simulink model "IEEE123_4subsystem"  (R2022b)
settings: Solver=ode4  StartTime=0.0  StopTime=inf  FixedStep=Ts  MaxStep=1e-4  RelTol=1e-3
PreLoadFcn:
  | Ts = 50e-6;
PostLoadFcn:
  | Ts = 50e-6;
InitFcn:
  | %%%%%%%%%%%%%%%%%%%%%%%%
  | % Simulation data for the IEEE 123 Node Test Feeder model
  | %%%%%%%%%%%%%%%%%%%%%%%
  | 
  | % miles/km
  | mi2km = 1.60934;
  | 
  | % feet to km
  | ft2km = 0.0003048;
  | 
  | % microsiemens to Farads
  | ms2F = 1/2/pi/60*1e-6;
  | 
  | %% Configuration 1 - series reactance - ohm/mile
  | 
  | R_1 = [0.4576 0.1560 0.1535;0.1560 0.4666 0.1580;0.1535 0.1580 0.4615];
  | X_1 = [1.0780 0.5017 0.3849;0.5017 1.0482 0.4236;0.3849 0.4236 1.0651];
  | 
  | % charging susceptance - microsiemens/mile
  | 
  | B_1 = [5.6765 -1.8319 -0.6982;-1.8319 5.9809 -1.1645;-0.6982 -1.1645 5.3971];
  | 
  | % convert for SPS
  | 
  | R_1 = R_1/mi2km;
  | 
  | Rs_1=(R_1(1,1)+R_1(2,2)+R_1(3,3))/3;
  | Rm_1=(R_1(1,2)+R_1(1,3)+R_1(2,3))/3;
  | R1_1=Rs_1-Rm_1;
  | R0_1=Rs_1+2*Rm_1;
  | 
  | L_1 = X_1/mi2km/2/pi/60;
  | 
  | Ls_1=(L_1(1,1)+L_1(2,2)+L_1(3,3))/3;
  | Lm_1=(L_1(1,2)+L_1(1,3)+L_1(2,3))/3;
  | L1_1=Ls_1-Lm_1;
  | L0_1=Ls_1+2*Lm_1;
  | 
  | C_1 = B_1/mi2km*ms2F;
  | 
  | Cs_1=(C_1(1,1)+C_1(2,2)+C_1(3,3))/3;
  | Cm_1=(C_1(1,2)+C_1(1,3)+C_1(2,3))/3;
  | C1_1=Cs_1-Cm_1;
  | C0_1=Cs_1+2*Cm_1;
  | 
  | 
  | %% Configuration 2 - series reactance - ohm/mile
  | 
  | R_2 = [0.4666 0.1580 0.1560;0.1580 0.4615 0.1535;0.1560 0.1535 0.4576];
  | X_2 = [1.0482 0.4236 0.5017;0.4236 1.0651 0.3849;0.5017 0.3849 1.0780];
  | 
  | % charging susceptance - microsiemens/mile
  | 
  | B_2 = [5.9809 -1.1645 -1.8319;-1.1645 5.3971 -0.6982;-1.8319 -0.6982 5.6765];
  | 
  | % convert for SPS
  | 
  | R_2 = R_2/mi2km;
  | 
  | Rs_2=(R_2(1,1)+R_2(2,2)+R_2(3,3))/3;
  | ... (+341 lines)
undefined symbols (not defined in the file): D1, Delta, find_system, I, Left, MOV_segment9, powergui, Right, type, V, X
libraries: spsGroundLib x242, spsThreePhaseVIMeasurementLib x134, spsSeriesRLCBranchLib x107, spsSeriesRLCLoadLib x83, spsPiSectionLineLib x61, spsThreePhasePISectionLineLib x60, spsVoltageMeasurementLib x52, spsDCVoltageSourceLib x36, ssn_lib x28, artemis x24, spsACCurrentSourceLib x18, spsOnDelayLib x18
(part 14 of 15)

== system IEEE123_4subsystem/SS_123p1/Regulator 4/Single Phase SVR_B/Transformer with Taps/SSN OLTC xfo v2/conn_down_d ==
  b2 : PMIOPort  Side=Right
  b1 : PMIOPort  Port=2  Side=Left
  connections:
  b1/RConn1 -- b2/RConn1

== system IEEE123_4subsystem/SS_123p1/Regulator 4/Single Phase SVR_B/Transformer with Taps/SSN OLTC xfo v2/conn_up_c ==
  b2 : PMIOPort  Side=Right
  b1 : PMIOPort  Port=2  Side=Left
  connections:
  b1/RConn1 -- b2/RConn1

== system IEEE123_4subsystem/SS_123p1/Regulator 4/Single Phase SVR_B/Transformer with Taps/SSN OLTC xfo v2/conn_up_d ==
  b2 : PMIOPort  Side=Right
  b1 : PMIOPort  Port=2  Side=Left
  connections:
  b1/RConn1 -- b2/RConn1

== system IEEE123_4subsystem/SS_123p1/Regulator 4/Single Phase SVR_B/Voltage Regulator Control/Tap Changer Control/Determine tap position ==
  NewTap : Inport
  Trigger : TriggerPort  VariantControl=Variant
  Memory : Memory  InitialCondition=InitialPosition  InheritSampleTime=on
  Saturation : Saturate  UpperLimit=MinMaxTap(2)  LowerLimit=MinMaxTap(1)
  Sum : Sum  Inputs=|++  SaturateOnIntegerOverflow=on
  TapNo : Outport  InitialOutput=InitialPosition  VectorParamsAs1DForOutWhenUnconnected=off
  wires:
  Saturation/1 -> Memory/1, TapNo/1
  Memory/1 -> Sum/2
  Sum/1 -> Saturation/1
  NewTap/1 -> Sum/1

== system IEEE123_4subsystem/SS_123p1/Regulator 4/Single Phase SVR_B/Voltage Regulator Control/Tap Changer Control/Edge Detector ==
  note: Edge or Slope Detector
  In : Inport
  Constant1 : Constant  Value=model
  Demux : Demux  Outputs=2
      settings: DisplayOption=none
  Logical Operator1 : Logic  Operator=OR
  Memory : Memory  InitialCondition=ic  LinearizeAsDelay=on
  Multiport Switch : MultiPortSwitch  InputSameDT=off
  NEGATIVE Edge : Subsystem  TreatAsAtomicUnit=on
  POSITIVE Edge : Subsystem  TreatAsAtomicUnit=on
  either edge : Constant  Value=[1 1]
  neg. edge : Constant  Value=[0 1]
  pos. edge : Constant  Value=[1 0]
  Out : Outport  VectorParamsAs1DForOutWhenUnconnected=off
  wires:
  Logical Operator1/1 -> Out/1
  NEGATIVE Edge/1(OUT) -> Logical Operator1/2
  POSITIVE Edge/1(OUT) -> Logical Operator1/1
  Memory/1 -> POSITIVE Edge/2(IN previous), NEGATIVE Edge/2(IN previous)
  In/1 -> POSITIVE Edge/1(IN), NEGATIVE Edge/1(IN), Memory/1
  pos. edge/1 -> Multiport Switch/2
  neg. edge/1 -> Multiport Switch/3
  Constant1/1 -> Multiport Switch/1
  Multiport Switch/1 -> Demux/1
  Demux/1 -> POSITIVE Edge/Enable
  Demux/2 -> NEGATIVE Edge/Enable
  either edge/1 -> Multiport Switch/4

== system IEEE123_4subsystem/SS_123p1/Regulator 4/Single Phase SVR_C/Transformer with Taps/SSN OLTC xfo v2/DC source_a ==
  I1A_V : spsDCVoltageSourceLib/DC Voltage Source  Amplitude=0  Measurements=None
  Conn1 : PMIOPort  Side=Left
  Conn2 : PMIOPort  Port=2  Side=Right
  connections:
  Conn1/RConn1 -- I1A_V/LConn1
  Conn2/RConn1 -- I1A_V/RConn1

== system IEEE123_4subsystem/SS_123p1/Regulator 4/Single Phase SVR_C/Transformer with Taps/SSN OLTC xfo v2/DC source_b ==
  I1B_V : spsDCVoltageSourceLib/DC Voltage Source  Amplitude=0  Measurements=None
  Conn3 : PMIOPort  Side=Left
  Conn4 : PMIOPort  Port=2  Side=Right
  connections:
  Conn4/RConn1 -- I1B_V/RConn1
  Conn3/RConn1 -- I1B_V/LConn1

== system IEEE123_4subsystem/SS_123p1/Regulator 4/Single Phase SVR_C/Transformer with Taps/SSN OLTC xfo v2/DC source_c ==
  I1C_V : spsDCVoltageSourceLib/DC Voltage Source  Amplitude=0  Measurements=None
  Conn1 : PMIOPort  Side=Left
  Conn2 : PMIOPort  Port=2  Side=Right
  connections:
  Conn2/RConn1 -- I1C_V/RConn1
  Conn1/RConn1 -- I1C_V/LConn1

== system IEEE123_4subsystem/SS_123p1/Regulator 4/Single Phase SVR_C/Transformer with Taps/SSN OLTC xfo v2/DC source_d ==
  I1D_V : spsDCVoltageSourceLib/DC Voltage Source  Amplitude=0  Measurements=None
  Conn3 : PMIOPort  Side=Left
  Conn4 : PMIOPort  Port=2  Side=Right
  connections:
  Conn3/RConn1 -- I1D_V/LConn1
  Conn4/RConn1 -- I1D_V/RConn1

== system IEEE123_4subsystem/SS_123p1/Regulator 4/Single Phase SVR_C/Transformer with Taps/SSN OLTC xfo v2/SSS-SM equations ==
  A : Inport
  B : Inport  Port=2
  C : Inport  Port=3
  u : Inport  Port=4
  Flux0 : Inport  Port=5
  Bphic : Inport  Port=6
  be : Inport  Port=7
  Constant : Constant
  Discretize : Subsystem
  Product{1..3,5..6} (5 alike) : Product  Multiplication=Matrix(*)  SaturateOnIntegerOverflow=on  OutDataTypeStr=Inherit: Same as first input
  Sum1 : Sum  Inputs=-+  SaturateOnIntegerOverflow=on
  Sum2 : Sum  Inputs=+++  SaturateOnIntegerOverflow=on
  Sum3 : Sum  SaturateOnIntegerOverflow=on
  mult1 : Product
  u5 : Constant  Value=eye(3,3)
  z-1 : UnitDelay  SampleTime=Ts  HasFrameUpgradeWarning=on
  Y : Outport  VectorParamsAs1DForOutWhenUnconnected=off
  Ihist : Outport  Port=2  VectorParamsAs1DForOutWhenUnconnected=off
  x : Outport  Port=3  VectorParamsAs1DForOutWhenUnconnected=off
  wires:
  u5/1 -> Discretize/3(Unity)
  Product2/1 -> Y/1
  A/1 -> Discretize/1(Ac)
  B/1 -> Discretize/2(Bc)
  C/1 -> Product2/1, Product6/1
  Product6/1 -> Ihist/1
  Product5/1 -> Sum3/2, mult1/1
  Product3/1 -> Sum2/1
  Sum3/1 -> Product3/2, x/1  "new_x"
  Sum2/1 -> z-1/1, Product6/2
  Discretize/1(Ad) -> Product3/1
  u/1 -> Product5/2
  z-1/1 -> Sum3/1
  Discretize/2(Bd) -> Product5/1, Product2/2
  Discretize/3(Bdin) -> Product1/1
  Product1/1 -> Sum2/3
  Flux0/1 -> Product1/2
  Bphic/1 -> Discretize/4(Bphic)
  Constant/1 -> Sum1/2
  mult1/1 -> Sum2/2
  Sum1/1 -> mult1/2  "=1 if trapeze           =0 if BE"
  be/1 -> Discretize/5(be), Sum1/1

== system IEEE123_4subsystem/SS_123p1/Regulator 4/Single Phase SVR_C/Transformer with Taps/SSN OLTC xfo v2/Update Matrix L ==
  k : Inport
  L2 : Inport  Port=2
  Lin : Inport  Port=3
  "L2->(2,2) " : Assignment  NumberOfDimensions=2  IndexOptions=Index vector (dialog),Index vector (dialog)  Indices=[2],[2]  OutputSizes=1,1
  k->(2,3) : Assignment  NumberOfDimensions=2  IndexOptions=Index vector (dialog),Index vector (dialog)  Indices=[2],[3]  OutputSizes=1,1
  L : Outport  VectorParamsAs1DForOutWhenUnconnected=off
  wires:
  "L2->(2,2) "/1 -> L/1
  L2/1 -> "L2->(2,2) "/2
  Lin/1 -> k->(2,3)/1
  k/1 -> k->(2,3)/2
  k->(2,3)/1 -> "L2->(2,2) "/1

== system IEEE123_4subsystem/SS_123p1/Regulator 4/Single Phase SVR_C/Transformer with Taps/SSN OLTC xfo v2/Update Matrix R ==
  R2 : Inport
  Rin : Inport  Port=2
  k : Inport  Port=3
  Rcore : Inport  Port=4
  Rcore/Lcore : Inport  Port=5
  "-R2->(2,2) " : Assignment  NumberOfDimensions=2  IndexOptions=Index vector (dialog),Index vector (dialog)  Indices=[2],[2]  OutputSizes=1,1
  -Rm/Lm->(3,3) : Assignment  NumberOfDimensions=2  IndexOptions=Index vector (dialog),Index vector (dialog)  Indices=3,3  OutputSizes=1,1
  Gain : Gain  Gain=-1
  Gain1 : Gain  Gain=-1
  Product1 : Product  RndMeth=Zero
  kRm->(3,2) : Assignment  NumberOfDimensions=2  IndexOptions=Index vector (dialog),Index vector (dialog)  Indices=3,2  OutputSizes=1,1
  R : Outport  VectorParamsAs1DForOutWhenUnconnected=off
  wires:
  "-R2->(2,2) "/1 -> kRm->(3,2)/1
  R2/1 -> Gain/1
  Rin/1 -> "-R2->(2,2) "/1
  Gain/1 -> "-R2->(2,2) "/2
  k/1 -> Product1/2
  Product1/1 -> kRm->(3,2)/2
  kRm->(3,2)/1 -> -Rm/Lm->(3,3)/1
  -Rm/Lm->(3,3)/1 -> R/1
  Rcore/1 -> Product1/1
  Gain1/1 -> -Rm/Lm->(3,3)/2
  Rcore/Lcore/1 -> Gain1/1

== system IEEE123_4subsystem/SS_123p1/Regulator 4/Single Phase SVR_C/Transformer with Taps/SSN OLTC xfo v2/conn_down_c ==
  b2 : PMIOPort  Side=Right
  b1 : PMIOPort  Port=2  Side=Left
  connections:
  b1/RConn1 -- b2/RConn1

== system IEEE123_4subsystem/SS_123p1/Regulator 4/Single Phase SVR_C/Transformer with Taps/SSN OLTC xfo v2/conn_down_d ==
  b2 : PMIOPort  Side=Right
  b1 : PMIOPort  Port=2  Side=Left
  connections:
  b1/RConn1 -- b2/RConn1

== system IEEE123_4subsystem/SS_123p1/Regulator 4/Single Phase SVR_C/Transformer with Taps/SSN OLTC xfo v2/conn_up_c ==
  b2 : PMIOPort  Side=Right
  b1 : PMIOPort  Port=2  Side=Left
  connections:
  b1/RConn1 -- b2/RConn1

== system IEEE123_4subsystem/SS_123p1/Regulator 4/Single Phase SVR_C/Transformer with Taps/SSN OLTC xfo v2/conn_up_d ==
  b2 : PMIOPort  Side=Right
  b1 : PMIOPort  Port=2  Side=Left
  connections:
  b1/RConn1 -- b2/RConn1

== system IEEE123_4subsystem/SS_123p1/Regulator 4/Single Phase SVR_C/Voltage Regulator Control/Tap Changer Control/Determine tap position ==
  NewTap : Inport
  Trigger : TriggerPort  VariantControl=Variant
  Memory : Memory  InitialCondition=InitialPosition  InheritSampleTime=on
  Saturation : Saturate  UpperLimit=MinMaxTap(2)  LowerLimit=MinMaxTap(1)
  Sum : Sum  Inputs=|++  SaturateOnIntegerOverflow=on
  TapNo : Outport  InitialOutput=InitialPosition  VectorParamsAs1DForOutWhenUnconnected=off
  wires:
  Saturation/1 -> Memory/1, TapNo/1
  Memory/1 -> Sum/2
  Sum/1 -> Saturation/1
  NewTap/1 -> Sum/1

== system IEEE123_4subsystem/SS_123p1/Regulator 4/Single Phase SVR_C/Voltage Regulator Control/Tap Changer Control/Edge Detector ==
  note: Edge or Slope Detector
  In : Inport
  Constant1 : Constant  Value=model
  Demux : Demux  Outputs=2
      settings: DisplayOption=none
  Logical Operator1 : Logic  Operator=OR
  Memory : Memory  InitialCondition=ic  LinearizeAsDelay=on
  Multiport Switch : MultiPortSwitch  InputSameDT=off
  NEGATIVE Edge : Subsystem  TreatAsAtomicUnit=on
  POSITIVE Edge : Subsystem  TreatAsAtomicUnit=on
  either edge : Constant  Value=[1 1]
  neg. edge : Constant  Value=[0 1]
  pos. edge : Constant  Value=[1 0]
  Out : Outport  VectorParamsAs1DForOutWhenUnconnected=off
  wires:
  Logical Operator1/1 -> Out/1
  NEGATIVE Edge/1(OUT) -> Logical Operator1/2
  POSITIVE Edge/1(OUT) -> Logical Operator1/1
  Memory/1 -> POSITIVE Edge/2(IN previous), NEGATIVE Edge/2(IN previous)
  In/1 -> POSITIVE Edge/1(IN), NEGATIVE Edge/1(IN), Memory/1
  pos. edge/1 -> Multiport Switch/2
  neg. edge/1 -> Multiport Switch/3
  Constant1/1 -> Multiport Switch/1
  Multiport Switch/1 -> Demux/1
  Demux/1 -> POSITIVE Edge/Enable
  Demux/2 -> NEGATIVE Edge/Enable
  either edge/1 -> Multiport Switch/4

== system IEEE123_4subsystem/SS_123p2/Regulator3/Single Phase SVR_A/Transformer with Taps/SSN OLTC xfo v2/DC source_a ==
  I1A_V : spsDCVoltageSourceLib/DC Voltage Source  Amplitude=0  Measurements=None
  Conn1 : PMIOPort  Side=Left
  Conn2 : PMIOPort  Port=2  Side=Right
  connections:
  Conn1/RConn1 -- I1A_V/LConn1
  Conn2/RConn1 -- I1A_V/RConn1

== system IEEE123_4subsystem/SS_123p2/Regulator3/Single Phase SVR_A/Transformer with Taps/SSN OLTC xfo v2/DC source_b ==
  I1B_V : spsDCVoltageSourceLib/DC Voltage Source  Amplitude=0  Measurements=None
  Conn3 : PMIOPort  Side=Left
  Conn4 : PMIOPort  Port=2  Side=Right
  connections:
  Conn4/RConn1 -- I1B_V/RConn1
  Conn3/RConn1 -- I1B_V/LConn1

== system IEEE123_4subsystem/SS_123p2/Regulator3/Single Phase SVR_A/Transformer with Taps/SSN OLTC xfo v2/DC source_c ==
  I1C_V : spsDCVoltageSourceLib/DC Voltage Source  Amplitude=0  Measurements=None
  Conn1 : PMIOPort  Side=Left
  Conn2 : PMIOPort  Port=2  Side=Right
  connections:
  Conn2/RConn1 -- I1C_V/RConn1
  Conn1/RConn1 -- I1C_V/LConn1

== system IEEE123_4subsystem/SS_123p2/Regulator3/Single Phase SVR_A/Transformer with Taps/SSN OLTC xfo v2/DC source_d ==
  I1D_V : spsDCVoltageSourceLib/DC Voltage Source  Amplitude=0  Measurements=None
  Conn3 : PMIOPort  Side=Left
  Conn4 : PMIOPort  Port=2  Side=Right
  connections:
  Conn3/RConn1 -- I1D_V/LConn1
  Conn4/RConn1 -- I1D_V/RConn1

== system IEEE123_4subsystem/SS_123p2/Regulator3/Single Phase SVR_A/Transformer with Taps/SSN OLTC xfo v2/SSS-SM equations ==
  A : Inport
  B : Inport  Port=2
  C : Inport  Port=3
  u : Inport  Port=4
  Flux0 : Inport  Port=5
  Bphic : Inport  Port=6
  be : Inport  Port=7
  Constant : Constant
  Discretize : Subsystem
  Product{1..3,5..6} (5 alike) : Product  Multiplication=Matrix(*)  SaturateOnIntegerOverflow=on  OutDataTypeStr=Inherit: Same as first input
  Sum1 : Sum  Inputs=-+  SaturateOnIntegerOverflow=on
  Sum2 : Sum  Inputs=+++  SaturateOnIntegerOverflow=on
  Sum3 : Sum  SaturateOnIntegerOverflow=on
  mult1 : Product
  u5 : Constant  Value=eye(3,3)
  z-1 : UnitDelay  SampleTime=Ts  HasFrameUpgradeWarning=on
  Y : Outport  VectorParamsAs1DForOutWhenUnconnected=off
  Ihist : Outport  Port=2  VectorParamsAs1DForOutWhenUnconnected=off
  x : Outport  Port=3  VectorParamsAs1DForOutWhenUnconnected=off
  wires:
  u5/1 -> Discretize/3(Unity)
  Product2/1 -> Y/1
  A/1 -> Discretize/1(Ac)
  B/1 -> Discretize/2(Bc)
  C/1 -> Product2/1, Product6/1
  Product6/1 -> Ihist/1
  Product5/1 -> Sum3/2, mult1/1
  Product3/1 -> Sum2/1
  Sum3/1 -> Product3/2, x/1  "new_x"
  Sum2/1 -> z-1/1, Product6/2
  Discretize/1(Ad) -> Product3/1
  u/1 -> Product5/2
  z-1/1 -> Sum3/1
  Discretize/2(Bd) -> Product5/1, Product2/2
  Discretize/3(Bdin) -> Product1/1
  Product1/1 -> Sum2/3
  Flux0/1 -> Product1/2
  Bphic/1 -> Discretize/4(Bphic)
  Constant/1 -> Sum1/2
  mult1/1 -> Sum2/2
  Sum1/1 -> mult1/2  "=1 if trapeze           =0 if BE"
  be/1 -> Discretize/5(be), Sum1/1

== system IEEE123_4subsystem/SS_123p2/Regulator3/Single Phase SVR_A/Transformer with Taps/SSN OLTC xfo v2/Update Matrix L ==
  k : Inport
  L2 : Inport  Port=2
  Lin : Inport  Port=3
  "L2->(2,2) " : Assignment  NumberOfDimensions=2  IndexOptions=Index vector (dialog),Index vector (dialog)  Indices=[2],[2]  OutputSizes=1,1
  k->(2,3) : Assignment  NumberOfDimensions=2  IndexOptions=Index vector (dialog),Index vector (dialog)  Indices=[2],[3]  OutputSizes=1,1
  L : Outport  VectorParamsAs1DForOutWhenUnconnected=off
  wires:
  "L2->(2,2) "/1 -> L/1
  L2/1 -> "L2->(2,2) "/2
  Lin/1 -> k->(2,3)/1
  k/1 -> k->(2,3)/2
  k->(2,3)/1 -> "L2->(2,2) "/1

== system IEEE123_4subsystem/SS_123p2/Regulator3/Single Phase SVR_A/Transformer with Taps/SSN OLTC xfo v2/Update Matrix R ==
  R2 : Inport
  Rin : Inport  Port=2
  k : Inport  Port=3
  Rcore : Inport  Port=4
  Rcore/Lcore : Inport  Port=5
  "-R2->(2,2) " : Assignment  NumberOfDimensions=2  IndexOptions=Index vector (dialog),Index vector (dialog)  Indices=[2],[2]  OutputSizes=1,1
  -Rm/Lm->(3,3) : Assignment  NumberOfDimensions=2  IndexOptions=Index vector (dialog),Index vector (dialog)  Indices=3,3  OutputSizes=1,1
  Gain : Gain  Gain=-1
  Gain1 : Gain  Gain=-1
  Product1 : Product  RndMeth=Zero
  kRm->(3,2) : Assignment  NumberOfDimensions=2  IndexOptions=Index vector (dialog),Index vector (dialog)  Indices=3,2  OutputSizes=1,1
  R : Outport  VectorParamsAs1DForOutWhenUnconnected=off
  wires:
  "-R2->(2,2) "/1 -> kRm->(3,2)/1
  R2/1 -> Gain/1
  Rin/1 -> "-R2->(2,2) "/1
  Gain/1 -> "-R2->(2,2) "/2
  k/1 -> Product1/2
  Product1/1 -> kRm->(3,2)/2
  kRm->(3,2)/1 -> -Rm/Lm->(3,3)/1
  -Rm/Lm->(3,3)/1 -> R/1
  Rcore/1 -> Product1/1
  Gain1/1 -> -Rm/Lm->(3,3)/2
  Rcore/Lcore/1 -> Gain1/1

== system IEEE123_4subsystem/SS_123p2/Regulator3/Single Phase SVR_A/Transformer with Taps/SSN OLTC xfo v2/conn_down_c ==
  b2 : PMIOPort  Side=Right
  b1 : PMIOPort  Port=2  Side=Left
  connections:
  b1/RConn1 -- b2/RConn1

== system IEEE123_4subsystem/SS_123p2/Regulator3/Single Phase SVR_A/Transformer with Taps/SSN OLTC xfo v2/conn_down_d ==
  b2 : PMIOPort  Side=Right
  b1 : PMIOPort  Port=2  Side=Left
  connections:
  b1/RConn1 -- b2/RConn1

== system IEEE123_4subsystem/SS_123p2/Regulator3/Single Phase SVR_A/Transformer with Taps/SSN OLTC xfo v2/conn_up_c ==
  b2 : PMIOPort  Side=Right
  b1 : PMIOPort  Port=2  Side=Left
  connections:
  b1/RConn1 -- b2/RConn1

== system IEEE123_4subsystem/SS_123p2/Regulator3/Single Phase SVR_A/Transformer with Taps/SSN OLTC xfo v2/conn_up_d ==
  b2 : PMIOPort  Side=Right
  b1 : PMIOPort  Port=2  Side=Left
  connections:
  b1/RConn1 -- b2/RConn1

== system IEEE123_4subsystem/SS_123p2/Regulator3/Single Phase SVR_A/Voltage Regulator Control/Tap Changer Control/Determine tap position ==
  NewTap : Inport
  Trigger : TriggerPort  VariantControl=Variant
  Memory : Memory  InitialCondition=InitialPosition  InheritSampleTime=on
  Saturation : Saturate  UpperLimit=MinMaxTap(2)  LowerLimit=MinMaxTap(1)
  Sum : Sum  Inputs=|++  SaturateOnIntegerOverflow=on
  TapNo : Outport  InitialOutput=InitialPosition  VectorParamsAs1DForOutWhenUnconnected=off
  wires:
  Saturation/1 -> Memory/1, TapNo/1
  Memory/1 -> Sum/2
  Sum/1 -> Saturation/1
  NewTap/1 -> Sum/1

== system IEEE123_4subsystem/SS_123p2/Regulator3/Single Phase SVR_A/Voltage Regulator Control/Tap Changer Control/Edge Detector ==
  note: Edge or Slope Detector
  In : Inport
  Constant1 : Constant  Value=model
  Demux : Demux  Outputs=2
      settings: DisplayOption=none
  Logical Operator1 : Logic  Operator=OR
  Memory : Memory  InitialCondition=ic  LinearizeAsDelay=on
  Multiport Switch : MultiPortSwitch  InputSameDT=off
  NEGATIVE Edge : Subsystem  TreatAsAtomicUnit=on
  POSITIVE Edge : Subsystem  TreatAsAtomicUnit=on
  either edge : Constant  Value=[1 1]
  neg. edge : Constant  Value=[0 1]
  pos. edge : Constant  Value=[1 0]
  Out : Outport  VectorParamsAs1DForOutWhenUnconnected=off
  wires:
  Logical Operator1/1 -> Out/1
  NEGATIVE Edge/1(OUT) -> Logical Operator1/2
  POSITIVE Edge/1(OUT) -> Logical Operator1/1
  Memory/1 -> POSITIVE Edge/2(IN previous), NEGATIVE Edge/2(IN previous)
  In/1 -> POSITIVE Edge/1(IN), NEGATIVE Edge/1(IN), Memory/1
  pos. edge/1 -> Multiport Switch/2
  neg. edge/1 -> Multiport Switch/3
  Constant1/1 -> Multiport Switch/1
  Multiport Switch/1 -> Demux/1
  Demux/1 -> POSITIVE Edge/Enable
  Demux/2 -> NEGATIVE Edge/Enable
  either edge/1 -> Multiport Switch/4

== system IEEE123_4subsystem/SS_123p2/Regulator3/Single Phase SVR_C/Transformer with Taps/SSN OLTC xfo v2/DC source_a ==
  I1A_V : spsDCVoltageSourceLib/DC Voltage Source  Amplitude=0  Measurements=None
  Conn1 : PMIOPort  Side=Left
  Conn2 : PMIOPort  Port=2  Side=Right
  connections:
  Conn1/RConn1 -- I1A_V/LConn1
  Conn2/RConn1 -- I1A_V/RConn1

== system IEEE123_4subsystem/SS_123p2/Regulator3/Single Phase SVR_C/Transformer with Taps/SSN OLTC xfo v2/DC source_b ==
  I1B_V : spsDCVoltageSourceLib/DC Voltage Source  Amplitude=0  Measurements=None
  Conn3 : PMIOPort  Side=Left
  Conn4 : PMIOPort  Port=2  Side=Right
  connections:
  Conn4/RConn1 -- I1B_V/RConn1
  Conn3/RConn1 -- I1B_V/LConn1

== system IEEE123_4subsystem/SS_123p2/Regulator3/Single Phase SVR_C/Transformer with Taps/SSN OLTC xfo v2/DC source_c ==
  I1C_V : spsDCVoltageSourceLib/DC Voltage Source  Amplitude=0  Measurements=None
  Conn1 : PMIOPort  Side=Left
  Conn2 : PMIOPort  Port=2  Side=Right
  connections:
  Conn2/RConn1 -- I1C_V/RConn1
  Conn1/RConn1 -- I1C_V/LConn1

== system IEEE123_4subsystem/SS_123p2/Regulator3/Single Phase SVR_C/Transformer with Taps/SSN OLTC xfo v2/DC source_d ==
  I1D_V : spsDCVoltageSourceLib/DC Voltage Source  Amplitude=0  Measurements=None
  Conn3 : PMIOPort  Side=Left
  Conn4 : PMIOPort  Port=2  Side=Right
  connections:
  Conn3/RConn1 -- I1D_V/LConn1
  Conn4/RConn1 -- I1D_V/RConn1

== system IEEE123_4subsystem/SS_123p2/Regulator3/Single Phase SVR_C/Transformer with Taps/SSN OLTC xfo v2/SSS-SM equations ==
  A : Inport
  B : Inport  Port=2
  C : Inport  Port=3
  u : Inport  Port=4
  Flux0 : Inport  Port=5
  Bphic : Inport  Port=6
  be : Inport  Port=7
  Constant : Constant
  Discretize : Subsystem
  Product{1..3,5..6} (5 alike) : Product  Multiplication=Matrix(*)  SaturateOnIntegerOverflow=on  OutDataTypeStr=Inherit: Same as first input
  Sum1 : Sum  Inputs=-+  SaturateOnIntegerOverflow=on
  Sum2 : Sum  Inputs=+++  SaturateOnIntegerOverflow=on
  Sum3 : Sum  SaturateOnIntegerOverflow=on
  mult1 : Product
  u5 : Constant  Value=eye(3,3)
  z-1 : UnitDelay  SampleTime=Ts  HasFrameUpgradeWarning=on
  Y : Outport  VectorParamsAs1DForOutWhenUnconnected=off
  Ihist : Outport  Port=2  VectorParamsAs1DForOutWhenUnconnected=off
  x : Outport  Port=3  VectorParamsAs1DForOutWhenUnconnected=off
  wires:
  u5/1 -> Discretize/3(Unity)
  Product2/1 -> Y/1
  A/1 -> Discretize/1(Ac)
  B/1 -> Discretize/2(Bc)
  C/1 -> Product2/1, Product6/1
  Product6/1 -> Ihist/1
  Product5/1 -> Sum3/2, mult1/1
  Product3/1 -> Sum2/1
  Sum3/1 -> Product3/2, x/1  "new_x"
  Sum2/1 -> z-1/1, Product6/2
  Discretize/1(Ad) -> Product3/1
  u/1 -> Product5/2
  z-1/1 -> Sum3/1
  Discretize/2(Bd) -> Product5/1, Product2/2
  Discretize/3(Bdin) -> Product1/1
  Product1/1 -> Sum2/3
  Flux0/1 -> Product1/2
  Bphic/1 -> Discretize/4(Bphic)
  Constant/1 -> Sum1/2
  mult1/1 -> Sum2/2
  Sum1/1 -> mult1/2  "=1 if trapeze           =0 if BE"
  be/1 -> Discretize/5(be), Sum1/1

== system IEEE123_4subsystem/SS_123p2/Regulator3/Single Phase SVR_C/Transformer with Taps/SSN OLTC xfo v2/Update Matrix L ==
  k : Inport
  L2 : Inport  Port=2
  Lin : Inport  Port=3
  "L2->(2,2) " : Assignment  NumberOfDimensions=2  IndexOptions=Index vector (dialog),Index vector (dialog)  Indices=[2],[2]  OutputSizes=1,1
  k->(2,3) : Assignment  NumberOfDimensions=2  IndexOptions=Index vector (dialog),Index vector (dialog)  Indices=[2],[3]  OutputSizes=1,1
  L : Outport  VectorParamsAs1DForOutWhenUnconnected=off
  wires:
  "L2->(2,2) "/1 -> L/1
  L2/1 -> "L2->(2,2) "/2
  Lin/1 -> k->(2,3)/1
  k/1 -> k->(2,3)/2
  k->(2,3)/1 -> "L2->(2,2) "/1

== system IEEE123_4subsystem/SS_123p2/Regulator3/Single Phase SVR_C/Transformer with Taps/SSN OLTC xfo v2/Update Matrix R ==
  R2 : Inport
  Rin : Inport  Port=2
  k : Inport  Port=3
  Rcore : Inport  Port=4
  Rcore/Lcore : Inport  Port=5
  "-R2->(2,2) " : Assignment  NumberOfDimensions=2  IndexOptions=Index vector (dialog),Index vector (dialog)  Indices=[2],[2]  OutputSizes=1,1
  -Rm/Lm->(3,3) : Assignment  NumberOfDimensions=2  IndexOptions=Index vector (dialog),Index vector (dialog)  Indices=3,3  OutputSizes=1,1
  Gain : Gain  Gain=-1
  Gain1 : Gain  Gain=-1
  Product1 : Product  RndMeth=Zero
  kRm->(3,2) : Assignment  NumberOfDimensions=2  IndexOptions=Index vector (dialog),Index vector (dialog)  Indices=3,2  OutputSizes=1,1
  R : Outport  VectorParamsAs1DForOutWhenUnconnected=off
  wires:
  "-R2->(2,2) "/1 -> kRm->(3,2)/1
  R2/1 -> Gain/1
  Rin/1 -> "-R2->(2,2) "/1
  Gain/1 -> "-R2->(2,2) "/2
  k/1 -> Product1/2
  Product1/1 -> kRm->(3,2)/2
  kRm->(3,2)/1 -> -Rm/Lm->(3,3)/1
  -Rm/Lm->(3,3)/1 -> R/1
  Rcore/1 -> Product1/1
  Gain1/1 -> -Rm/Lm->(3,3)/2
  Rcore/Lcore/1 -> Gain1/1

== system IEEE123_4subsystem/SS_123p2/Regulator3/Single Phase SVR_C/Transformer with Taps/SSN OLTC xfo v2/conn_down_c ==
  b2 : PMIOPort  Side=Right
  b1 : PMIOPort  Port=2  Side=Left
  connections:
  b1/RConn1 -- b2/RConn1

== system IEEE123_4subsystem/SS_123p2/Regulator3/Single Phase SVR_C/Transformer with Taps/SSN OLTC xfo v2/conn_down_d ==
  b2 : PMIOPort  Side=Right
  b1 : PMIOPort  Port=2  Side=Left
  connections:
  b1/RConn1 -- b2/RConn1

== system IEEE123_4subsystem/SS_123p2/Regulator3/Single Phase SVR_C/Transformer with Taps/SSN OLTC xfo v2/conn_up_c ==
  b2 : PMIOPort  Side=Right
  b1 : PMIOPort  Port=2  Side=Left
  connections:
  b1/RConn1 -- b2/RConn1

== system IEEE123_4subsystem/SS_123p2/Regulator3/Single Phase SVR_C/Transformer with Taps/SSN OLTC xfo v2/conn_up_d ==
  b2 : PMIOPort  Side=Right
  b1 : PMIOPort  Port=2  Side=Left
  connections:
  b1/RConn1 -- b2/RConn1

== system IEEE123_4subsystem/SS_123p2/Regulator3/Single Phase SVR_C/Voltage Regulator Control/Tap Changer Control/Determine tap position ==
  NewTap : Inport
  Trigger : TriggerPort  VariantControl=Variant
  Memory : Memory  InitialCondition=InitialPosition  InheritSampleTime=on
  Saturation : Saturate  UpperLimit=MinMaxTap(2)  LowerLimit=MinMaxTap(1)
  Sum : Sum  Inputs=|++  SaturateOnIntegerOverflow=on
  TapNo : Outport  InitialOutput=InitialPosition  VectorParamsAs1DForOutWhenUnconnected=off
  wires:
  Saturation/1 -> Memory/1, TapNo/1
  Memory/1 -> Sum/2
  Sum/1 -> Saturation/1
  NewTap/1 -> Sum/1

== system IEEE123_4subsystem/SS_123p2/Regulator3/Single Phase SVR_C/Voltage Regulator Control/Tap Changer Control/Edge Detector ==
  note: Edge or Slope Detector
  In : Inport
  Constant1 : Constant  Value=model
  Demux : Demux  Outputs=2
      settings: DisplayOption=none
  Logical Operator1 : Logic  Operator=OR
  Memory : Memory  InitialCondition=ic  LinearizeAsDelay=on
  Multiport Switch : MultiPortSwitch  InputSameDT=off
  NEGATIVE Edge : Subsystem  TreatAsAtomicUnit=on
  POSITIVE Edge : Subsystem  TreatAsAtomicUnit=on
  either edge : Constant  Value=[1 1]
  neg. edge : Constant  Value=[0 1]
  pos. edge : Constant  Value=[1 0]
  Out : Outport  VectorParamsAs1DForOutWhenUnconnected=off
  wires:
  Logical Operator1/1 -> Out/1
  NEGATIVE Edge/1(OUT) -> Logical Operator1/2
  POSITIVE Edge/1(OUT) -> Logical Operator1/1
  Memory/1 -> POSITIVE Edge/2(IN previous), NEGATIVE Edge/2(IN previous)
  In/1 -> POSITIVE Edge/1(IN), NEGATIVE Edge/1(IN), Memory/1
  pos. edge/1 -> Multiport Switch/2
  neg. edge/1 -> Multiport Switch/3
  Constant1/1 -> Multiport Switch/1
  Multiport Switch/1 -> Demux/1
  Demux/1 -> POSITIVE Edge/Enable
  Demux/2 -> NEGATIVE Edge/Enable
  either edge/1 -> Multiport Switch/4

== system IEEE123_4subsystem/SM_123p/Regulator 1 Three Phase Ganged SVR/Single Phase SVR_A/Transformer with Taps/SSN OLTC xfo v2/SSS-SM equations/Discretize ==
  Ac : Inport
  Bc : Inport  Port=2
  Unity : Inport  Port=3
  Bphic : Inport  Port=4
  be : Inport  Port=5
  Bias : Bias  Bias=1  SaturateOnIntegerOverflow=off
  Constant : Constant
  Product1 : Product  Multiplication=Matrix(*)  SaturateOnIntegerOverflow=on  OutDataTypeStr=Inherit: Same as first input
  Product2 : Product  Multiplication=Matrix(*)  SaturateOnIntegerOverflow=on  OutDataTypeStr=Inherit: Same as first input
  Product4 : Product  Multiplication=Matrix(*)  SaturateOnIntegerOverflow=on  OutDataTypeStr=Inherit: Same as first input
  Sum1 : Sum  Inputs=+-  SaturateOnIntegerOverflow=on
  Sum2 : Sum  Inputs=-+  SaturateOnIntegerOverflow=on
  Sum5 : Sum  SaturateOnIntegerOverflow=on
  Ts/2 : Gain  Gain=Ts/2  SaturateOnIntegerOverflow=on  OutDataTypeStr=Inherit: Same as input  ParamDataTypeStr=Inherit: Same as input
  inversion : Product  Inputs=/  Multiplication=Matrix(*)  RndMeth=Zero
  mult : Product
  mult1 : Product
  mult2 : Product
  trapeze has Ts/2 factor on B : Gain  Gain=Ts/2  SaturateOnIntegerOverflow=on  OutDataTypeStr=Inherit: Same as input  ParamDataTypeStr=Inherit: Same as input
  trapeze has Ts/2 factor on B1 : Gain  Gain=Ts  SaturateOnIntegerOverflow=on  OutDataTypeStr=Inherit: Same as input  ParamDataTypeStr=Inherit: Same as input
  Ad : Outport  VectorParamsAs1DForOutWhenUnconnected=off
  Bd : Outport  Port=2  VectorParamsAs1DForOutWhenUnconnected=off
  Bdin : Outport  Port=3  VectorParamsAs1DForOutWhenUnconnected=off
  wires:
  Sum1/1 -> inversion/1
  Ac/1 -> Ts/2/1
  Product1/1 -> Bd/1
  Sum5/1 -> Product4/2
  Unity/1 -> Sum1/1, Sum5/1
  Product4/1 -> Ad/1
  Ts/2/1 -> mult/1
  Bc/1 -> trapeze has Ts/2 factor on B/1
  inversion/1 -> Product4/1, Product1/1, Product2/1  "inv(I4-Ts/2*A)"
  Product2/1 -> Bdin/1
  trapeze has Ts/2 factor on B1/1 -> Product2/2
  Bphic/1 -> trapeze has Ts/2 factor on B1/1
  mult/1 -> Sum1/2, mult2/1
  be/1 -> Bias/1, Sum2/1
  Bias/1 -> mult/2, mult1/2
  trapeze has Ts/2 factor on B/1 -> mult1/1
  mult1/1 -> Product1/2
  mult2/1 -> Sum5/2
  Constant/1 -> Sum2/2
  Sum2/1 -> mult2/2

== system IEEE123_4subsystem/SM_123p/Regulator 1 Three Phase Ganged SVR/Single Phase SVR_A/Voltage Regulator Control/Tap Changer Control/Edge Detector/NEGATIVE Edge ==
  IN : Inport
  IN previous : Inport  Port=2
  Enable : EnablePort  PropagateVarSize=During execution
  Relational Operator1 : RelationalOperator  Operator=>
  OUT : Outport  VectorParamsAs1DForOutWhenUnconnected=off
  wires:
  Relational Operator1/1 -> OUT/1
  IN previous/1 -> Relational Operator1/1
  IN/1 -> Relational Operator1/2

== system IEEE123_4subsystem/SM_123p/Regulator 1 Three Phase Ganged SVR/Single Phase SVR_A/Voltage Regulator Control/Tap Changer Control/Edge Detector/POSITIVE Edge ==
  IN : Inport
  IN previous : Inport  Port=2
  Enable : EnablePort  PropagateVarSize=During execution
  Relational Operator1 : RelationalOperator  Operator=>
  OUT : Outport  VectorParamsAs1DForOutWhenUnconnected=off
  wires:
  Relational Operator1/1 -> OUT/1
  IN previous/1 -> Relational Operator1/2
  IN/1 -> Relational Operator1/1

== system IEEE123_4subsystem/SM_123p/Regulator 1 Three Phase Ganged SVR/Single Phase SVR_B/Transformer with Taps/SSN OLTC xfo v2/SSS-SM equations/Discretize ==
  Ac : Inport
  Bc : Inport  Port=2
  Unity : Inport  Port=3
  Bphic : Inport  Port=4
  be : Inport  Port=5
  Bias : Bias  Bias=1  SaturateOnIntegerOverflow=off
  Constant : Constant
  Product1 : Product  Multiplication=Matrix(*)  SaturateOnIntegerOverflow=on  OutDataTypeStr=Inherit: Same as first input
  Product2 : Product  Multiplication=Matrix(*)  SaturateOnIntegerOverflow=on  OutDataTypeStr=Inherit: Same as first input
  Product4 : Product  Multiplication=Matrix(*)  SaturateOnIntegerOverflow=on  OutDataTypeStr=Inherit: Same as first input
  Sum1 : Sum  Inputs=+-  SaturateOnIntegerOverflow=on
  Sum2 : Sum  Inputs=-+  SaturateOnIntegerOverflow=on
  Sum5 : Sum  SaturateOnIntegerOverflow=on
  Ts/2 : Gain  Gain=Ts/2  SaturateOnIntegerOverflow=on  OutDataTypeStr=Inherit: Same as input  ParamDataTypeStr=Inherit: Same as input
  inversion : Product  Inputs=/  Multiplication=Matrix(*)  RndMeth=Zero
  mult : Product
  mult1 : Product
  mult2 : Product
  trapeze has Ts/2 factor on B : Gain  Gain=Ts/2  SaturateOnIntegerOverflow=on  OutDataTypeStr=Inherit: Same as input  ParamDataTypeStr=Inherit: Same as input
  trapeze has Ts/2 factor on B1 : Gain  Gain=Ts  SaturateOnIntegerOverflow=on  OutDataTypeStr=Inherit: Same as input  ParamDataTypeStr=Inherit: Same as input
  Ad : Outport  VectorParamsAs1DForOutWhenUnconnected=off
  Bd : Outport  Port=2  VectorParamsAs1DForOutWhenUnconnected=off
  Bdin : Outport  Port=3  VectorParamsAs1DForOutWhenUnconnected=off
  wires:
  Sum1/1 -> inversion/1
  Ac/1 -> Ts/2/1
  Product1/1 -> Bd/1
  Sum5/1 -> Product4/2
  Unity/1 -> Sum1/1, Sum5/1
  Product4/1 -> Ad/1
  Ts/2/1 -> mult/1
  Bc/1 -> trapeze has Ts/2 factor on B/1
  inversion/1 -> Product4/1, Product1/1, Product2/1  "inv(I4-Ts/2*A)"
  Product2/1 -> Bdin/1
  trapeze has Ts/2 factor on B1/1 -> Product2/2
  Bphic/1 -> trapeze has Ts/2 factor on B1/1
  mult/1 -> Sum1/2, mult2/1
  be/1 -> Bias/1, Sum2/1
  Bias/1 -> mult/2, mult1/2
  trapeze has Ts/2 factor on B/1 -> mult1/1
  mult1/1 -> Product1/2
  mult2/1 -> Sum5/2
  Constant/1 -> Sum2/2
  Sum2/1 -> mult2/2

== system IEEE123_4subsystem/SM_123p/Regulator 1 Three Phase Ganged SVR/Single Phase SVR_B/Voltage Regulator Control/Tap Changer Control/Edge Detector/NEGATIVE Edge ==
  IN : Inport
  IN previous : Inport  Port=2
  Enable : EnablePort  PropagateVarSize=During execution
  Relational Operator1 : RelationalOperator  Operator=>
  OUT : Outport  VectorParamsAs1DForOutWhenUnconnected=off
  wires:
  Relational Operator1/1 -> OUT/1
  IN previous/1 -> Relational Operator1/1
  IN/1 -> Relational Operator1/2

== system IEEE123_4subsystem/SM_123p/Regulator 1 Three Phase Ganged SVR/Single Phase SVR_B/Voltage Regulator Control/Tap Changer Control/Edge Detector/POSITIVE Edge ==
  IN : Inport
  IN previous : Inport  Port=2
  Enable : EnablePort  PropagateVarSize=During execution
  Relational Operator1 : RelationalOperator  Operator=>
  OUT : Outport  VectorParamsAs1DForOutWhenUnconnected=off
  wires:
  Relational Operator1/1 -> OUT/1
  IN previous/1 -> Relational Operator1/2
  IN/1 -> Relational Operator1/1

== system IEEE123_4subsystem/SM_123p/Regulator 1 Three Phase Ganged SVR/Single Phase SVR_C/Transformer with Taps/SSN OLTC xfo v2/SSS-SM equations/Discretize ==
  Ac : Inport
  Bc : Inport  Port=2
  Unity : Inport  Port=3
  Bphic : Inport  Port=4
  be : Inport  Port=5
  Bias : Bias  Bias=1  SaturateOnIntegerOverflow=off
  Constant : Constant
  Product1 : Product  Multiplication=Matrix(*)  SaturateOnIntegerOverflow=on  OutDataTypeStr=Inherit: Same as first input
  Product2 : Product  Multiplication=Matrix(*)  SaturateOnIntegerOverflow=on  OutDataTypeStr=Inherit: Same as first input
  Product4 : Product  Multiplication=Matrix(*)  SaturateOnIntegerOverflow=on  OutDataTypeStr=Inherit: Same as first input
  Sum1 : Sum  Inputs=+-  SaturateOnIntegerOverflow=on
  Sum2 : Sum  Inputs=-+  SaturateOnIntegerOverflow=on
  Sum5 : Sum  SaturateOnIntegerOverflow=on
  Ts/2 : Gain  Gain=Ts/2  SaturateOnIntegerOverflow=on  OutDataTypeStr=Inherit: Same as input  ParamDataTypeStr=Inherit: Same as input
  inversion : Product  Inputs=/  Multiplication=Matrix(*)  RndMeth=Zero
  mult : Product
  mult1 : Product
  mult2 : Product
  trapeze has Ts/2 factor on B : Gain  Gain=Ts/2  SaturateOnIntegerOverflow=on  OutDataTypeStr=Inherit: Same as input  ParamDataTypeStr=Inherit: Same as input
  trapeze has Ts/2 factor on B1 : Gain  Gain=Ts  SaturateOnIntegerOverflow=on  OutDataTypeStr=Inherit: Same as input  ParamDataTypeStr=Inherit: Same as input
  Ad : Outport  VectorParamsAs1DForOutWhenUnconnected=off
  Bd : Outport  Port=2  VectorParamsAs1DForOutWhenUnconnected=off
  Bdin : Outport  Port=3  VectorParamsAs1DForOutWhenUnconnected=off
  wires:
  Sum1/1 -> inversion/1
  Ac/1 -> Ts/2/1
  Product1/1 -> Bd/1
  Sum5/1 -> Product4/2
  Unity/1 -> Sum1/1, Sum5/1
  Product4/1 -> Ad/1
  Ts/2/1 -> mult/1
  Bc/1 -> trapeze has Ts/2 factor on B/1
  inversion/1 -> Product4/1, Product1/1, Product2/1  "inv(I4-Ts/2*A)"
  Product2/1 -> Bdin/1
  trapeze has Ts/2 factor on B1/1 -> Product2/2
  Bphic/1 -> trapeze has Ts/2 factor on B1/1
  mult/1 -> Sum1/2, mult2/1
  be/1 -> Bias/1, Sum2/1
  Bias/1 -> mult/2, mult1/2
  trapeze has Ts/2 factor on B/1 -> mult1/1
  mult1/1 -> Product1/2
  mult2/1 -> Sum5/2
  Constant/1 -> Sum2/2
  Sum2/1 -> mult2/2

== system IEEE123_4subsystem/SM_123p/Regulator 1 Three Phase Ganged SVR/Single Phase SVR_C/Voltage Regulator Control/Tap Changer Control/Edge Detector/NEGATIVE Edge ==
  IN : Inport
  IN previous : Inport  Port=2
  Enable : EnablePort  PropagateVarSize=During execution
  Relational Operator1 : RelationalOperator  Operator=>
  OUT : Outport  VectorParamsAs1DForOutWhenUnconnected=off
  wires:
  Relational Operator1/1 -> OUT/1
  IN previous/1 -> Relational Operator1/1
  IN/1 -> Relational Operator1/2

== system IEEE123_4subsystem/SM_123p/Regulator 1 Three Phase Ganged SVR/Single Phase SVR_C/Voltage Regulator Control/Tap Changer Control/Edge Detector/POSITIVE Edge ==
  IN : Inport
  IN previous : Inport  Port=2
  Enable : EnablePort  PropagateVarSize=During execution
  Relational Operator1 : RelationalOperator  Operator=>
  OUT : Outport  VectorParamsAs1DForOutWhenUnconnected=off
  wires:
  Relational Operator1/1 -> OUT/1
  IN previous/1 -> Relational Operator1/2
  IN/1 -> Relational Operator1/1

== system IEEE123_4subsystem/SM_123p/Regulator 2/Single Phase SVR_A/Transformer with Taps/SSN OLTC xfo v2/SSS-SM equations/Discretize ==
  Ac : Inport
  Bc : Inport  Port=2
  Unity : Inport  Port=3
  Bphic : Inport  Port=4
  be : Inport  Port=5
  Bias : Bias  Bias=1  SaturateOnIntegerOverflow=off
  Constant : Constant
  Product1 : Product  Multiplication=Matrix(*)  SaturateOnIntegerOverflow=on  OutDataTypeStr=Inherit: Same as first input
  Product2 : Product  Multiplication=Matrix(*)  SaturateOnIntegerOverflow=on  OutDataTypeStr=Inherit: Same as first input
  Product4 : Product  Multiplication=Matrix(*)  SaturateOnIntegerOverflow=on  OutDataTypeStr=Inherit: Same as first input
  Sum1 : Sum  Inputs=+-  SaturateOnIntegerOverflow=on
  Sum2 : Sum  Inputs=-+  SaturateOnIntegerOverflow=on
  Sum5 : Sum  SaturateOnIntegerOverflow=on
  Ts/2 : Gain  Gain=Ts/2  SaturateOnIntegerOverflow=on  OutDataTypeStr=Inherit: Same as input  ParamDataTypeStr=Inherit: Same as input
  inversion : Product  Inputs=/  Multiplication=Matrix(*)  RndMeth=Zero
  mult : Product
  mult1 : Product
  mult2 : Product
  trapeze has Ts/2 factor on B : Gain  Gain=Ts/2  SaturateOnIntegerOverflow=on  OutDataTypeStr=Inherit: Same as input  ParamDataTypeStr=Inherit: Same as input
  trapeze has Ts/2 factor on B1 : Gain  Gain=Ts  SaturateOnIntegerOverflow=on  OutDataTypeStr=Inherit: Same as input  ParamDataTypeStr=Inherit: Same as input
  Ad : Outport  VectorParamsAs1DForOutWhenUnconnected=off
  Bd : Outport  Port=2  VectorParamsAs1DForOutWhenUnconnected=off
  Bdin : Outport  Port=3  VectorParamsAs1DForOutWhenUnconnected=off
  wires:
  Sum1/1 -> inversion/1
  Ac/1 -> Ts/2/1
  Product1/1 -> Bd/1
  Sum5/1 -> Product4/2
  Unity/1 -> Sum1/1, Sum5/1
  Product4/1 -> Ad/1
  Ts/2/1 -> mult/1
  Bc/1 -> trapeze has Ts/2 factor on B/1
  inversion/1 -> Product4/1, Product1/1, Product2/1  "inv(I4-Ts/2*A)"
  Product2/1 -> Bdin/1
  trapeze has Ts/2 factor on B1/1 -> Product2/2
  Bphic/1 -> trapeze has Ts/2 factor on B1/1
  mult/1 -> Sum1/2, mult2/1
  be/1 -> Bias/1, Sum2/1
  Bias/1 -> mult/2, mult1/2
  trapeze has Ts/2 factor on B/1 -> mult1/1
  mult1/1 -> Product1/2
  mult2/1 -> Sum5/2
  Constant/1 -> Sum2/2
  Sum2/1 -> mult2/2

== system IEEE123_4subsystem/SM_123p/Regulator 2/Single Phase SVR_A/Voltage Regulator Control/Tap Changer Control/Edge Detector/NEGATIVE Edge ==
  IN : Inport
  IN previous : Inport  Port=2
  Enable : EnablePort  PropagateVarSize=During execution
  Relational Operator1 : RelationalOperator  Operator=>
  OUT : Outport  VectorParamsAs1DForOutWhenUnconnected=off
  wires:
  Relational Operator1/1 -> OUT/1
  IN previous/1 -> Relational Operator1/1
  IN/1 -> Relational Operator1/2

== system IEEE123_4subsystem/SM_123p/Regulator 2/Single Phase SVR_A/Voltage Regulator Control/Tap Changer Control/Edge Detector/POSITIVE Edge ==
  IN : Inport
  IN previous : Inport  Port=2
  Enable : EnablePort  PropagateVarSize=During execution
  Relational Operator1 : RelationalOperator  Operator=>
  OUT : Outport  VectorParamsAs1DForOutWhenUnconnected=off
  wires:
  Relational Operator1/1 -> OUT/1
  IN previous/1 -> Relational Operator1/2
  IN/1 -> Relational Operator1/1

== system IEEE123_4subsystem/SS_123p1/Regulator 4/Single Phase SVR_A/Transformer with Taps/SSN OLTC xfo v2/SSS-SM equations/Discretize ==
  Ac : Inport
  Bc : Inport  Port=2
  Unity : Inport  Port=3
  Bphic : Inport  Port=4
  be : Inport  Port=5
  Bias : Bias  Bias=1  SaturateOnIntegerOverflow=off
  Constant : Constant
  Product1 : Product  Multiplication=Matrix(*)  SaturateOnIntegerOverflow=on  OutDataTypeStr=Inherit: Same as first input
  Product2 : Product  Multiplication=Matrix(*)  SaturateOnIntegerOverflow=on  OutDataTypeStr=Inherit: Same as first input
  Product4 : Product  Multiplication=Matrix(*)  SaturateOnIntegerOverflow=on  OutDataTypeStr=Inherit: Same as first input
  Sum1 : Sum  Inputs=+-  SaturateOnIntegerOverflow=on
  Sum2 : Sum  Inputs=-+  SaturateOnIntegerOverflow=on
  Sum5 : Sum  SaturateOnIntegerOverflow=on
  Ts/2 : Gain  Gain=Ts/2  SaturateOnIntegerOverflow=on  OutDataTypeStr=Inherit: Same as input  ParamDataTypeStr=Inherit: Same as input
  inversion : Product  Inputs=/  Multiplication=Matrix(*)  RndMeth=Zero
  mult : Product
  mult1 : Product
  mult2 : Product
  trapeze has Ts/2 factor on B : Gain  Gain=Ts/2  SaturateOnIntegerOverflow=on  OutDataTypeStr=Inherit: Same as input  ParamDataTypeStr=Inherit: Same as input
  trapeze has Ts/2 factor on B1 : Gain  Gain=Ts  SaturateOnIntegerOverflow=on  OutDataTypeStr=Inherit: Same as input  ParamDataTypeStr=Inherit: Same as input
  Ad : Outport  VectorParamsAs1DForOutWhenUnconnected=off
  Bd : Outport  Port=2  VectorParamsAs1DForOutWhenUnconnected=off
  Bdin : Outport  Port=3  VectorParamsAs1DForOutWhenUnconnected=off
  wires:
  Sum1/1 -> inversion/1
  Ac/1 -> Ts/2/1
  Product1/1 -> Bd/1
  Sum5/1 -> Product4/2
  Unity/1 -> Sum1/1, Sum5/1
  Product4/1 -> Ad/1
  Ts/2/1 -> mult/1
  Bc/1 -> trapeze has Ts/2 factor on B/1
  inversion/1 -> Product4/1, Product1/1, Product2/1  "inv(I4-Ts/2*A)"
  Product2/1 -> Bdin/1
  trapeze has Ts/2 factor on B1/1 -> Product2/2
  Bphic/1 -> trapeze has Ts/2 factor on B1/1
  mult/1 -> Sum1/2, mult2/1
  be/1 -> Bias/1, Sum2/1
  Bias/1 -> mult/2, mult1/2
  trapeze has Ts/2 factor on B/1 -> mult1/1
  mult1/1 -> Product1/2
  mult2/1 -> Sum5/2
  Constant/1 -> Sum2/2
  Sum2/1 -> mult2/2

== system IEEE123_4subsystem/SS_123p1/Regulator 4/Single Phase SVR_A/Voltage Regulator Control/Tap Changer Control/Edge Detector/NEGATIVE Edge ==
  IN : Inport
  IN previous : Inport  Port=2
  Enable : EnablePort  PropagateVarSize=During execution
  Relational Operator1 : RelationalOperator  Operator=>
  OUT : Outport  VectorParamsAs1DForOutWhenUnconnected=off
  wires:
  Relational Operator1/1 -> OUT/1
  IN previous/1 -> Relational Operator1/1
  IN/1 -> Relational Operator1/2

== system IEEE123_4subsystem/SS_123p1/Regulator 4/Single Phase SVR_A/Voltage Regulator Control/Tap Changer Control/Edge Detector/POSITIVE Edge ==
  IN : Inport
  IN previous : Inport  Port=2
  Enable : EnablePort  PropagateVarSize=During execution
  Relational Operator1 : RelationalOperator  Operator=>
  OUT : Outport  VectorParamsAs1DForOutWhenUnconnected=off
  wires:
  Relational Operator1/1 -> OUT/1
  IN previous/1 -> Relational Operator1/2
  IN/1 -> Relational Operator1/1

== system IEEE123_4subsystem/SS_123p1/Regulator 4/Single Phase SVR_B/Transformer with Taps/SSN OLTC xfo v2/SSS-SM equations/Discretize ==
  Ac : Inport
  Bc : Inport  Port=2
  Unity : Inport  Port=3
  Bphic : Inport  Port=4
  be : Inport  Port=5
  Bias : Bias  Bias=1  SaturateOnIntegerOverflow=off
  Constant : Constant
  Product1 : Product  Multiplication=Matrix(*)  SaturateOnIntegerOverflow=on  OutDataTypeStr=Inherit: Same as first input
  Product2 : Product  Multiplication=Matrix(*)  SaturateOnIntegerOverflow=on  OutDataTypeStr=Inherit: Same as first input
  Product4 : Product  Multiplication=Matrix(*)  SaturateOnIntegerOverflow=on  OutDataTypeStr=Inherit: Same as first input
  Sum1 : Sum  Inputs=+-  SaturateOnIntegerOverflow=on
  Sum2 : Sum  Inputs=-+  SaturateOnIntegerOverflow=on
  Sum5 : Sum  SaturateOnIntegerOverflow=on
  Ts/2 : Gain  Gain=Ts/2  SaturateOnIntegerOverflow=on  OutDataTypeStr=Inherit: Same as input  ParamDataTypeStr=Inherit: Same as input
  inversion : Product  Inputs=/  Multiplication=Matrix(*)  RndMeth=Zero
  mult : Product
  mult1 : Product
  mult2 : Product
  trapeze has Ts/2 factor on B : Gain  Gain=Ts/2  SaturateOnIntegerOverflow=on  OutDataTypeStr=Inherit: Same as input  ParamDataTypeStr=Inherit: Same as input
  trapeze has Ts/2 factor on B1 : Gain  Gain=Ts  SaturateOnIntegerOverflow=on  OutDataTypeStr=Inherit: Same as input  ParamDataTypeStr=Inherit: Same as input
  Ad : Outport  VectorParamsAs1DForOutWhenUnconnected=off
  Bd : Outport  Port=2  VectorParamsAs1DForOutWhenUnconnected=off
  Bdin : Outport  Port=3  VectorParamsAs1DForOutWhenUnconnected=off
  wires:
  Sum1/1 -> inversion/1
  Ac/1 -> Ts/2/1
  Product1/1 -> Bd/1
  Sum5/1 -> Product4/2
  Unity/1 -> Sum1/1, Sum5/1
  Product4/1 -> Ad/1
  Ts/2/1 -> mult/1
  Bc/1 -> trapeze has Ts/2 factor on B/1
  inversion/1 -> Product4/1, Product1/1, Product2/1  "inv(I4-Ts/2*A)"
  Product2/1 -> Bdin/1
  trapeze has Ts/2 factor on B1/1 -> Product2/2
  Bphic/1 -> trapeze has Ts/2 factor on B1/1
  mult/1 -> Sum1/2, mult2/1
  be/1 -> Bias/1, Sum2/1
  Bias/1 -> mult/2, mult1/2
  trapeze has Ts/2 factor on B/1 -> mult1/1
  mult1/1 -> Product1/2
  mult2/1 -> Sum5/2
  Constant/1 -> Sum2/2
  Sum2/1 -> mult2/2

== system IEEE123_4subsystem/SS_123p1/Regulator 4/Single Phase SVR_B/Voltage Regulator Control/Tap Changer Control/Edge Detector/NEGATIVE Edge ==
  IN : Inport
  IN previous : Inport  Port=2
  Enable : EnablePort  PropagateVarSize=During execution
  Relational Operator1 : RelationalOperator  Operator=>
  OUT : Outport  VectorParamsAs1DForOutWhenUnconnected=off
  wires:
  Relational Operator1/1 -> OUT/1
  IN previous/1 -> Relational Operator1/1
  IN/1 -> Relational Operator1/2

== system IEEE123_4subsystem/SS_123p1/Regulator 4/Single Phase SVR_B/Voltage Regulator Control/Tap Changer Control/Edge Detector/POSITIVE Edge ==
  IN : Inport
  IN previous : Inport  Port=2
  Enable : EnablePort  PropagateVarSize=During execution
  Relational Operator1 : RelationalOperator  Operator=>
  OUT : Outport  VectorParamsAs1DForOutWhenUnconnected=off
  wires:
  Relational Operator1/1 -> OUT/1
  IN previous/1 -> Relational Operator1/2
  IN/1 -> Relational Operator1/1

== system IEEE123_4subsystem/SS_123p1/Regulator 4/Single Phase SVR_C/Transformer with Taps/SSN OLTC xfo v2/SSS-SM equations/Discretize ==
  Ac : Inport
  Bc : Inport  Port=2
  Unity : Inport  Port=3
  Bphic : Inport  Port=4
  be : Inport  Port=5
  Bias : Bias  Bias=1  SaturateOnIntegerOverflow=off
  Constant : Constant
  Product1 : Product  Multiplication=Matrix(*)  SaturateOnIntegerOverflow=on  OutDataTypeStr=Inherit: Same as first input
  Product2 : Product  Multiplication=Matrix(*)  SaturateOnIntegerOverflow=on  OutDataTypeStr=Inherit: Same as first input
  Product4 : Product  Multiplication=Matrix(*)  SaturateOnIntegerOverflow=on  OutDataTypeStr=Inherit: Same as first input
  Sum1 : Sum  Inputs=+-  SaturateOnIntegerOverflow=on
  Sum2 : Sum  Inputs=-+  SaturateOnIntegerOverflow=on
  Sum5 : Sum  SaturateOnIntegerOverflow=on
  Ts/2 : Gain  Gain=Ts/2  SaturateOnIntegerOverflow=on  OutDataTypeStr=Inherit: Same as input  ParamDataTypeStr=Inherit: Same as input
  inversion : Product  Inputs=/  Multiplication=Matrix(*)  RndMeth=Zero
  mult : Product
  mult1 : Product
  mult2 : Product
  trapeze has Ts/2 factor on B : Gain  Gain=Ts/2  SaturateOnIntegerOverflow=on  OutDataTypeStr=Inherit: Same as input  ParamDataTypeStr=Inherit: Same as input
  trapeze has Ts/2 factor on B1 : Gain  Gain=Ts  SaturateOnIntegerOverflow=on  OutDataTypeStr=Inherit: Same as input  ParamDataTypeStr=Inherit: Same as input
  Ad : Outport  VectorParamsAs1DForOutWhenUnconnected=off
  Bd : Outport  Port=2  VectorParamsAs1DForOutWhenUnconnected=off
  Bdin : Outport  Port=3  VectorParamsAs1DForOutWhenUnconnected=off
  wires:
  Sum1/1 -> inversion/1
  Ac/1 -> Ts/2/1
  Product1/1 -> Bd/1
  Sum5/1 -> Product4/2
  Unity/1 -> Sum1/1, Sum5/1
  Product4/1 -> Ad/1
  Ts/2/1 -> mult/1
  Bc/1 -> trapeze has Ts/2 factor on B/1
  inversion/1 -> Product4/1, Product1/1, Product2/1  "inv(I4-Ts/2*A)"
  Product2/1 -> Bdin/1
  trapeze has Ts/2 factor on B1/1 -> Product2/2
  Bphic/1 -> trapeze has Ts/2 factor on B1/1
  mult/1 -> Sum1/2, mult2/1
  be/1 -> Bias/1, Sum2/1
  Bias/1 -> mult/2, mult1/2
  trapeze has Ts/2 factor on B/1 -> mult1/1
  mult1/1 -> Product1/2
  mult2/1 -> Sum5/2
  Constant/1 -> Sum2/2
  Sum2/1 -> mult2/2

== system IEEE123_4subsystem/SS_123p1/Regulator 4/Single Phase SVR_C/Voltage Regulator Control/Tap Changer Control/Edge Detector/NEGATIVE Edge ==
  IN : Inport
  IN previous : Inport  Port=2
  Enable : EnablePort  PropagateVarSize=During execution
  Relational Operator1 : RelationalOperator  Operator=>
  OUT : Outport  VectorParamsAs1DForOutWhenUnconnected=off
  wires:
  Relational Operator1/1 -> OUT/1
  IN previous/1 -> Relational Operator1/1
  IN/1 -> Relational Operator1/2

== system IEEE123_4subsystem/SS_123p1/Regulator 4/Single Phase SVR_C/Voltage Regulator Control/Tap Changer Control/Edge Detector/POSITIVE Edge ==
  IN : Inport
  IN previous : Inport  Port=2
  Enable : EnablePort  PropagateVarSize=During execution
  Relational Operator1 : RelationalOperator  Operator=>
  OUT : Outport  VectorParamsAs1DForOutWhenUnconnected=off
  wires:
  Relational Operator1/1 -> OUT/1
  IN previous/1 -> Relational Operator1/2
  IN/1 -> Relational Operator1/1
